simulink model "buck_pid_config"  (R2019b)
settings: Solver=VariableStepAuto  StartTime=0.0  StopTime=10.0  RelTol=1e-3
settings Model: Creator=khduh  LastModifiedBy=khduh

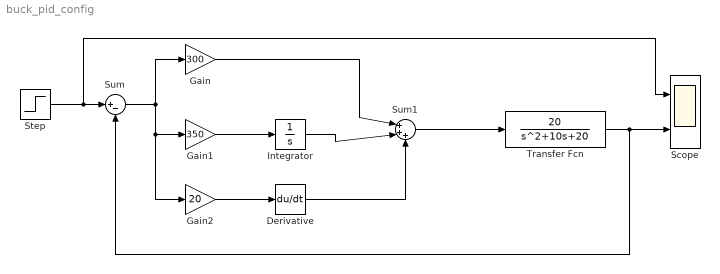
== system buck_pid_config ==
  Derivative : Derivative
  Gain : Gain  Gain=300
  Gain1 : Gain  Gain=350
  Gain2 : Gain  Gain=20
  Integrator : Integrator
  Scope : Scope  NumInputPorts=2
  Step : Step  SampleTime=0
  Sum : Sum  Inputs=|+-
  Sum1 : Sum  Inputs=|+++
  Transfer Fcn : TransferFcn  Numerator=[20]  Denominator=[1 10 20]
  wires:
  Step/1 -> Scope/1, Sum/1
  Gain1/1 -> Integrator/1
  Gain2/1 -> Derivative/1
  Integrator/1 -> Sum1/2
  Derivative/1 -> Sum1/3
  Gain/1 -> Sum1/1
  Sum1/1 -> Transfer Fcn/1
  Transfer Fcn/1 -> Scope/2, Sum/2
  Sum/1 -> Gain2/1, Gain1/1, Gain/1
